simulink model "ekstraLoopSimu"  (R2015a)
settings: Solver=ode3  StartTime=0.0  StopTime=50  FixedStep=.01  RelTol=1e-3
values from neighbouring files (symbols this model uses):
  s = tf('s')    [ekstranul.m]
undefined symbols (not defined in the file or in its folder): B, g, jp, l, mp
libraries: cstblocks x6, simulink x2
settings Model: Creator=morten  LastModifiedBy=morten

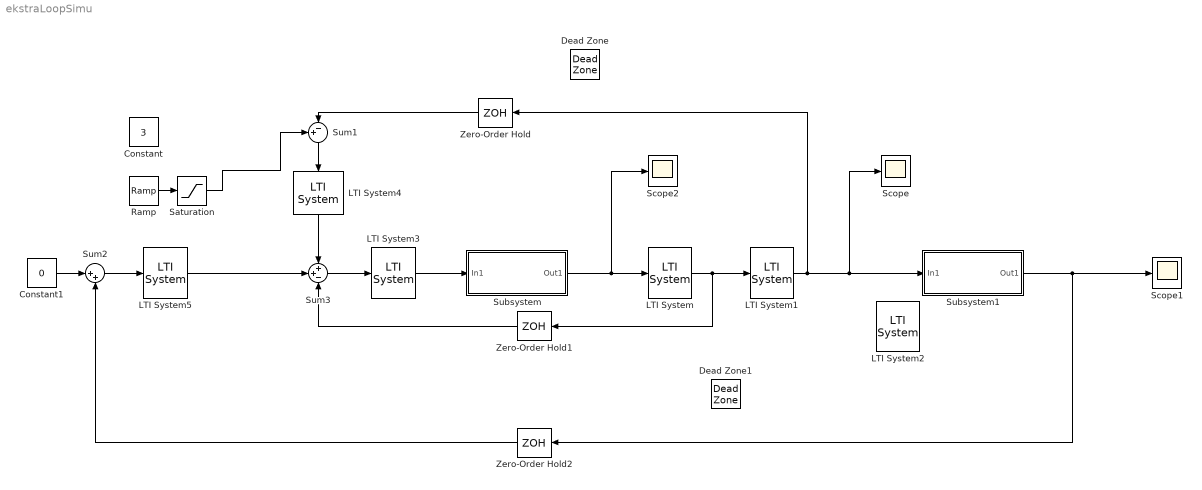
== system ekstraLoopSimu ==
  Constant : Constant  Value=3
  Constant1 : Constant  Value=0
  Dead Zone : DeadZone  LowerValue=-0.005  UpperValue=0.005  SaturateOnIntegerOverflow=on
  Dead Zone1 : DeadZone  LowerValue=-0.001  UpperValue=0.001  SaturateOnIntegerOverflow=on
  LTI System : cstblocks/LTI System  sys=Hv  IC=[]
  LTI System1 : cstblocks/LTI System  sys=1/s  IC=[]
  LTI System2 : cstblocks/LTI System  sys=W  IC=[]
  LTI System3 : cstblocks/LTI System  sys=C1  IC=[]
  LTI System4 : cstblocks/LTI System  sys=C2  IC=[]
  LTI System5 : cstblocks/LTI System  sys=dC3  IC=[]
  Ramp : simulink/Sources/Ramp  slope=.5  start=0  X0=0
  Saturation : Saturate  UpperLimit=3  LowerLimit=0
  Scope : Scope
  Scope1 : Scope
  Scope2 : Scope
      settings: SaveName=ScopeData2
  Subsystem : Subsystem
  Subsystem1 : Subsystem
  Sum1 : Sum  Inputs=+-|
  Sum2 : Sum  Inputs=|++
  Sum3 : Sum  Inputs=++-
  Zero-Order Hold : ZeroOrderHold  SampleTime=.01
  Zero-Order Hold1 : ZeroOrderHold  SampleTime=.01
  Zero-Order Hold2 : ZeroOrderHold  SampleTime=.01
  wires:
  Sum2/1 -> LTI System5/1
  Sum1/1 -> LTI System4/1
  Saturation/1 -> Sum1/1
  Constant1/1 -> Sum2/1
  LTI System3/1 -> Subsystem/1(In1)
  LTI System1/1 -> Subsystem1/1(In1), Scope/1, Zero-Order Hold/1
  Subsystem1/1(Out1) -> Scope1/1, Zero-Order Hold2/1
  Ramp/1 -> Saturation/1
  LTI System4/1 -> Sum3/1
  LTI System5/1 -> Sum3/2
  Sum3/1 -> LTI System3/1
  LTI System/1 -> Zero-Order Hold1/1, LTI System1/1
  Subsystem/1(Out1) -> Scope2/1, LTI System/1
  Zero-Order Hold2/1 -> Sum2/2
  Zero-Order Hold1/1 -> Sum3/3
  Zero-Order Hold/1 -> Sum1/2

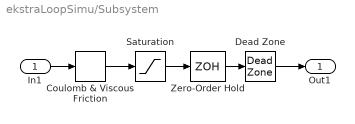
== system ekstraLoopSimu/Subsystem ==
  In1 : Inport
  Coulomb & Viscous Friction : simulink/Discontinuities/Coulomb & Viscous Friction  offset=[4.5]  gain=1
  Dead Zone : DeadZone  LowerValue=-4.5  UpperValue=4.5  SaturateOnIntegerOverflow=on
  Saturation : Saturate  UpperLimit=12.5  LowerLimit=-12.5
  Zero-Order Hold : ZeroOrderHold  SampleTime=.01
  Out1 : Outport
  wires:
  In1/1 -> Coulomb & Viscous Friction/1
  Zero-Order Hold/1 -> Dead Zone/1
  Saturation/1 -> Zero-Order Hold/1
  Coulomb & Viscous Friction/1 -> Saturation/1
  Dead Zone/1 -> Out1/1

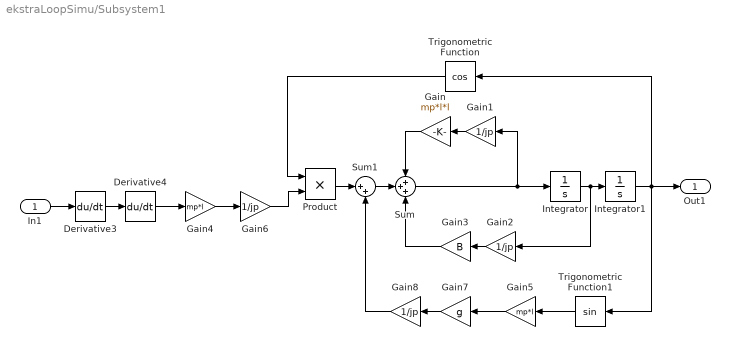
== system ekstraLoopSimu/Subsystem1 ==
  In1 : Inport
  Derivative3 : Derivative
  Derivative4 : Derivative
  Gain : Gain  Gain=mp*l*l
  Gain{1..2,6,8} (4 alike) : Gain  Gain=1/jp
  Gain3 : Gain  Gain=B
  Gain4 : Gain  Gain=mp*l
  Gain5 : Gain  Gain=mp*l
  Gain7 : Gain  Gain=g
  Integrator : Integrator
  Integrator1 : Integrator
  Product : Product
  Sum : Sum  Inputs=+++
  Sum1 : Sum  Inputs=|++
  Trigonometric Function : Trigonometry  Operator=cos
  Trigonometric Function1 : Trigonometry
  Out1 : Outport
  wires:
  Sum/1 -> Gain1/1, Integrator/1
  Integrator/1 -> Gain2/1, Integrator1/1
  Gain/1 -> Sum/1
  Gain1/1 -> Gain/1
  Gain2/1 -> Gain3/1
  Gain3/1 -> Sum/3
  Integrator1/1 -> Trigonometric Function1/1, Trigonometric Function/1, Out1/1
  In1/1 -> Derivative3/1
  Derivative3/1 -> Derivative4/1
  Derivative4/1 -> Gain4/1
  Product/1 -> Sum1/1
  Trigonometric Function/1 -> Product/1
  Gain4/1 -> Gain6/1
  Gain6/1 -> Product/2
  Trigonometric Function1/1 -> Gain5/1
  Gain5/1 -> Gain7/1
  Gain7/1 -> Gain8/1
  Gain8/1 -> Sum1/2
  Sum1/1 -> Sum/2
